simulink model "main_commande_PID"  (R2024b)
settings: Solver=FixedStepAuto  StartTime=0.0  StopTime=10.0  MaxStep=0.01  RelTol=1e-3
libraries: simulink x2
settings Model: PacingRate=0.100000  Creator=marti  LastModifiedBy=Filip

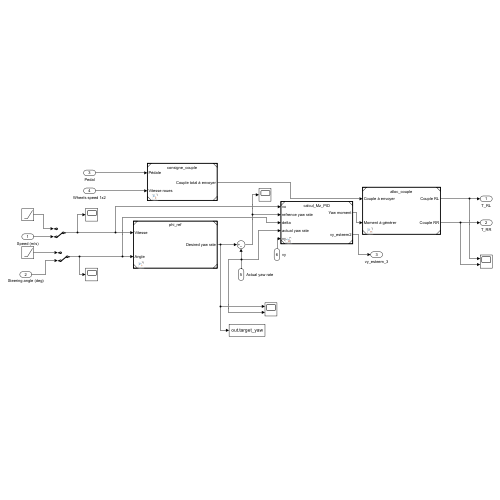
[thumbnail: Simulink's stored preview of the top-level diagram]
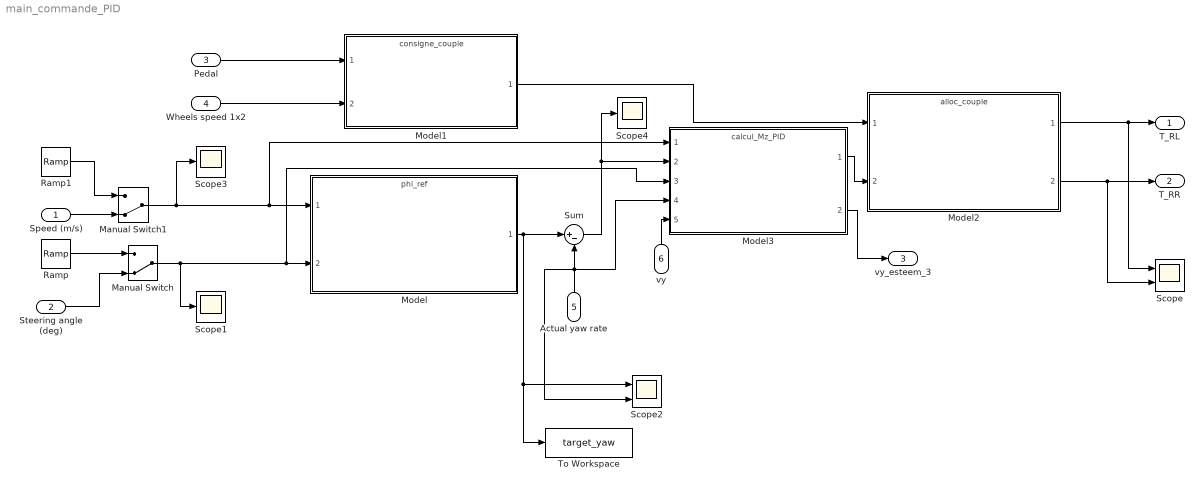
== system main_commande_PID ==
  Speed (m/s) : Inport
  Steering angle (deg) : Inport  Port=2
  Pedal : Inport  Port=3
  Wheels speed 1x2 : Inport  Port=4
  Actual yaw rate : Inport  Port=5
  vy : Inport  Port=6
  Manual Switch : ManualSwitch  CurrentSetting=0
  Manual Switch1 : ManualSwitch  CurrentSetting=0
  Model : ModelReference  ModelNameDialog=phi_ref.slx  SimulationMode=Normal  ModelReferenceVersion=1.22
  Model1 : ModelReference  ModelNameDialog=consigne_couple.slx  SimulationMode=Normal  ModelReferenceVersion=1.13
  Model2 : ModelReference  ModelNameDialog=alloc_couple.slx  SimulationMode=Normal  ModelReferenceVersion=1.5
  Model3 : ModelReference  ModelNameDialog=calcul_Mz_PID.slx  SimulationMode=Normal  ModelReferenceVersion=1.25
  Ramp : simulink/Sources/Ramp  slope=5  start=2  InitialOutput=0
  Ramp1 : simulink/Sources/Ramp  slope=10  start=0  InitialOutput=1
  Scope : Scope  NumInputPorts=2
  Scope1 : Scope
  Scope2 : Scope  NumInputPorts=2
  Scope3 : Scope
  Scope4 : Scope
  Sum : Sum  Inputs=|+-
  To Workspace : ToWorkspace  VariableName=target_yaw  SaveFormat=Structure With Time  SampleTime=-1
  T_RL : Outport
  T_RR : Outport  Port=2
  vy_esteem_3 : Outport  Port=3
  wires:
  Model3/1 -> Model2/2
  Pedal/1 -> Model1/1
  Wheels speed 1x2/1 -> Model1/2
  Model1/1 -> Model2/1
  Model2/1 -> Scope/1, T_RL/1
  Model2/2 -> Scope/2, T_RR/1
  Manual Switch/1 -> Scope1/1, Model3/3, Model/2
  Ramp/1 -> Manual Switch/1
  Steering angle (deg)/1 -> Manual Switch/2
  Manual Switch1/1 -> Scope3/1, Model/1, Model3/1
  Speed (m/s)/1 -> Manual Switch1/2
  Ramp1/1 -> Manual Switch1/1
  Model/1 -> Sum/1, To Workspace/1, Scope2/1
  Sum/1 -> Scope4/1, Model3/2
  Actual yaw rate/1 -> Sum/2, Model3/4, Scope2/2
  vy/1 -> Model3/5
  Model3/2 -> vy_esteem_3/1
